simulink model "zvysovaci_menic"  (Simulink 8.0)
settings: Solver=ode3  StartTime=0.0  StopTime=0.1  FixedStep=1e-6  RelTol=1e-3
undefined symbols (not defined in the file): plecsedit
libraries: simulink x1
settings Model: Creator=dragounj  LastModifiedBy=Kasi
settings DataIOCC: SignalLoggingSaveFormat=ModelDataLogs
settings DebuggingCC: FcnCallInpInsideContextMsg=UseLocalSettings
settings GRTTargetCC: CombineOutputUpdateFcns=off  GRTInterface=on

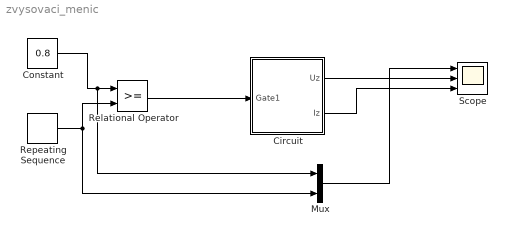
== system zvysovaci_menic ==
  Circuit : Subsystem  LoadFcn=plecsedit('sl', 200);  InitFcn=plecsedit('sl', 214);  StartFcn=plecsedit('sl', 208);  StopFcn=plecsedit('sl', 209);  mask(PlecsCircuit){}
      mask init:
      | % PLACE CUSTOM INITIALIZATIONS ABOVE
      | % DO NOT REMOVE
      | plecsedit('sl', 215);
      | % DO NOT REMOVE
      settings: CopyFcn=plecsedit('sl', 203);  DeleteFcn=plecsedit('sl', 205);  UndoDeleteFcn=plecsedit('sl', 206);  PreSaveFcn=plecsedit('sl', 211);  PostSaveFcn=plecsedit('sl', 201);  NameChangeFcn=plecsedit('sl', 210);  DestroyFcn=plecsedit('sl', 207);  PreCopyFcn=plecsedit('sl', 216);  OpenFcn=plecsedit('sl', 202);  ErrorFcn=plerrorfcn
      mask Display: disp('PLECS\nCircuit')
  Constant : Constant  Value=0.8
  Mux : Mux  Inputs=2
  Relational Operator : RelationalOperator  OutDataTypeStr=boolean
  Repeating Sequence : simulink/Sources/Repeating Sequence  rep_seq_t=[0 0.5 1]/1000  rep_seq_y=[0 1 0]
  Scope : Scope  NumInputPorts=3
      settings: YMin=-5~-5~-5  YMax=5~5~5
  wires:
  Constant/1 -> Relational Operator/1, Mux/1
  Repeating Sequence/1 -> Relational Operator/2, Mux/2
  Relational Operator/1 -> Circuit/1(Gate1)
  Mux/1 -> Scope/1
  Circuit/1(Uz) -> Scope/2
  Circuit/2(Iz) -> Scope/3

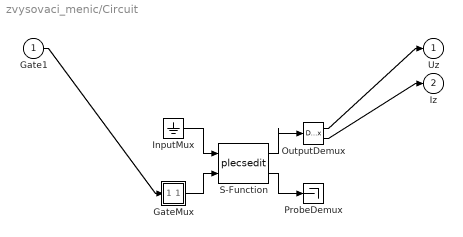
== system zvysovaci_menic/Circuit ==
  Gate1 : Inport  PortDimensions=1
  " GateMux " : Subsystem
      mask Display: disp('Mux')
  " InputMux " : Ground
  " OutputDemux " : Demux  Outputs=[ 1 1 ]
  " ProbeDemux " : Terminator
  " S-Function " : S-Function  FunctionName=plecsedit  EnableBusSupport=off
  Uz : Outport  PortDimensions=1
  Iz : Outport  Port=2  PortDimensions=1
  wires:
  " S-Function "/1 -> " OutputDemux "/1
  " InputMux "/1 -> " S-Function "/1
  " GateMux "/1(Out) -> " S-Function "/2
  " S-Function "/2 -> " ProbeDemux "/1
  Gate1/1 -> " GateMux "/1(In1)
  " OutputDemux "/1 -> Uz/1
  " OutputDemux "/2 -> Iz/1

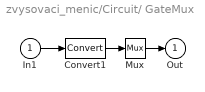
== system zvysovaci_menic/Circuit/ GateMux  ==
  In1 : Inport
  Convert1 : DataTypeConversion  SaturateOnIntegerOverflow=on  RndMeth=Zero
  Mux : Mux  Inputs=[ 1 ]
  Out : Outport
  wires:
  Mux/1 -> Out/1
  In1/1 -> Convert1/1
  Convert1/1 -> Mux/1
